simulink model "cubli_3d_model_quaternions2023"  (R2023a)
settings: Solver=ode4  StartTime=0.0  StopTime=10  FixedStep=0.01  RelTol=1e-3
InitFcn:
  | cubli_3d_model_quaternion_init
values from neighbouring files (symbols this model uses):
  b = 0    [cubli_3d_model_quaternion_init.m]
  bw = 1.06e-5    (= 1.06e-05)    [cubli_3d_model_quaternion_init.m]
  g = [0;0;9.81]    [cubli_3d_model_quaternion_init.m]
  GAMMA = [1 1 -1 0; 1 -1 0 1; -1 0 -1 1; 0 1 1 1]    [cubli_3d_model_quaternion_init.m]
  Ic_line = (Is_O + Iw1_O + Iw2_O + Iw3_O) - Iw    [cubli_3d_model_quaternion_init.m]
  invV = [0 0 0 1; 0 0 1 0; 0 -1 0 0; -1 0 0 0]    [cubli_3d_model_quaternion_init.m]
  Iw = [Iw_xx 0 0; 0 Iw_xx 0; 0 0 Iw_xx]    [cubli_3d_model_quaternion_init.m]
  l = 0.15    [cubli_3d_model_quaternion_init.m]
  mc_line = ms + 2*mw    (= 0.7)    [cubli_3d_model_quaternion_init.m]
  qs_init = [sqrt(2/3*(3-sqrt(3)))/2, -sqrt(1/3*(3+sqrt(3)))/2, sqrt(1/3*(3+sqrt(3)))/2, 0]'    [cubli_3d_model_quaternion_init.m]
  tauc = 2.46e-3    (= 0.00246)    [cubli_3d_model_quaternion_init.m]
libraries: simulink x1, matrix_library x1
settings Model: Creator=dozav  LastModifiedBy=dozav
settings RTWCC: GPUComputeCapability=5.0
settings ConfigComp: CovBoundaryAbsTol=1.0e-5

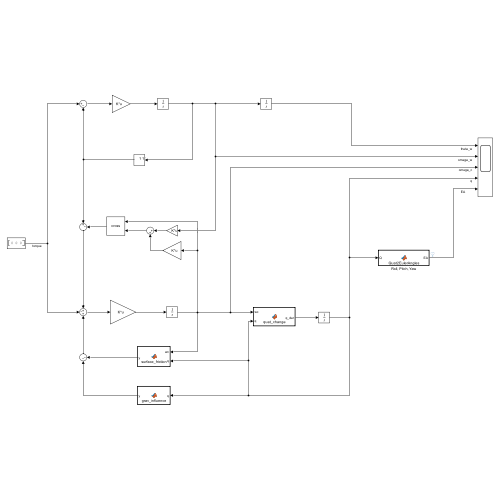
[thumbnail: Simulink's stored preview of the top-level diagram]
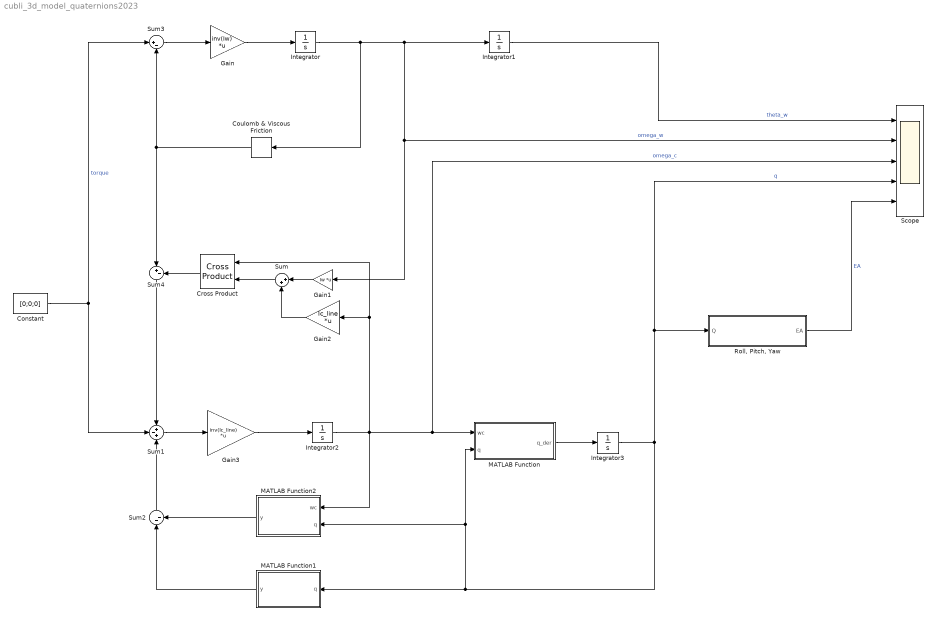
== system cubli_3d_model_quaternions2023 ==
  Constant : Constant  Value=[0;0;0]
  Coulomb & Viscous Friction : simulink/Discontinuities/Coulomb & Viscous Friction  offset=[tauc tauc tauc]  gain=[bw bw bw]
  Cross Product : matrix_library/Cross Product
  Gain : Gain  Gain=inv(Iw)  Multiplication=Matrix(K*u)
  Gain1 : Gain  Gain=Iw  Multiplication=Matrix(K*u)
  Gain2 : Gain  Gain=Ic_line  Multiplication=Matrix(K*u)
  Gain3 : Gain  Gain=inv(Ic_line)  Multiplication=Matrix(K*u)
  Integrator : Integrator  InitialCondition=[0; 0; 0]
  Integrator1 : Integrator  InitialCondition=[0; 0; 0]
  Integrator2 : Integrator  InitialCondition=[0; 0; 0]
  Integrator3 : Integrator  InitialCondition=qs_init
  MATLAB Function : MATLAB Function  TreatAsAtomicUnit=on
  MATLAB Function1 : MATLAB Function  TreatAsAtomicUnit=on
  MATLAB Function2 : MATLAB Function  TreatAsAtomicUnit=on
  "Roll, Pitch, Yaw" : MATLAB Function  TreatAsAtomicUnit=on
  Scope : Scope  NumInputPorts=5
  Sum : Sum  Inputs=|++
  Sum1 : Sum  Inputs=+-+
  Sum2 : Sum  Inputs=|--
  Sum3 : Sum  Inputs=|+-
  Sum4 : Sum  Inputs=|+-
  wires:
  Gain/1 -> Integrator/1
  Gain1/1 -> Sum/1
  Gain2/1 -> Sum/2
  Sum/1 -> Cross Product/2
  Integrator2/1 -> MATLAB Function2/1(wc), Gain2/1, Cross Product/1, Scope/3, MATLAB Function/1(wc)  "omega_c"
  Gain3/1 -> Integrator2/1
  Sum1/1 -> Gain3/1
  Constant/1 -> Sum3/1, Sum1/2  "torque"
  Sum2/1 -> Sum1/3
  Sum3/1 -> Gain/1
  Cross Product/1 -> Sum4/2
  Sum4/1 -> Sum1/1
  Integrator3/1 -> "Roll, Pitch, Yaw"/1(Q), Scope/4, MATLAB Function/2(q), MATLAB Function2/2(q), MATLAB Function1/1(q)  "q"
  MATLAB Function/1(q_der) -> Integrator3/1
  MATLAB Function1/1(y) -> Sum2/1
  Integrator/1 -> Coulomb & Viscous Friction/1, Gain1/1, Scope/2, Integrator1/1  "omega_w"
  Integrator1/1 -> Scope/1  "theta_w"
  Coulomb & Viscous Friction/1 -> Sum3/2, Sum4/1
  MATLAB Function2/1(y) -> Sum2/2
  "Roll, Pitch, Yaw"/1(EA) -> Scope/5  "EA"

== matlab function cubli_3d_model_quaternions2023/MATLAB Function1 ==
  data: q input; y output; GAMMA parameter; l parameter; g parameter; mc_line parameter
function y = grav_influence(q, GAMMA, l, g, mc_line)
%#codegen

q_skew = [0 -q(4) q(3); q(4) 0 -q(2); -q(3) q(2) 0];
G = [-q(2:4) q(1)*eye(3,3)-q_skew];

y = mc_line*9.81*l*(G*GAMMA*q);

== matlab function cubli_3d_model_quaternions2023/MATLAB Function ==
  data: wc input; q input; q_der output
function q_der = quat_change(wc, q)
%#codegen

q_skew = [0 -q(4) q(3); q(4) 0 -q(2); -q(3) q(2) 0];
G = [-q(2:4) q(1)*eye(3,3)-q_skew];

q_der = 1/2*G'*wc;

== matlab function cubli_3d_model_quaternions2023/MATLAB Function2 ==
  data: wc input; q input; y output; invV parameter; b parameter
function y = surface_friction(wc, q, invV, b)
%#codegen

q_skew = [0 -q(4) q(3); q(4) 0 -q(2); -q(3) q(2) 0];
G = [-q(2:4) q(1)*eye(3,3)-q_skew];




y = b*(G*invV*q*(G*invV*q)')*wc;

== matlab function cubli_3d_model_quaternions2023/Roll, Pitch, Yaw ==
  settings: sampleTime=0.1
  data: Q input; EA output
function EA  = Quat2EulerAngles(Q)

% Q = normr(Q);

% q0 = Q(1);
% q1 = Q(2);
% q2 = Q(3);
% q3 = Q(4);
% 
% EA = [atan2d(-2*(q2.*q3 - q1.*q0), q0.^2 - q1.^2 - q2.^2 + q3.^2), ...
%     asind(2*(q1.*q3 + q2.*q0)), ...
%     atan2d(-2*(q1.*q2 - q3.*q0), q0.^2 + q1.^2 - q2.^2 - q3.^2)];

Q = Q/norm(Q);

qw = Q(1);
qx = Q(2);
qy = Q(3);
qz = Q(4);

EA = [atan2d(2*(qw*qx+qy*qz),1-2*(qx^2+qy^2)); asind(2*(qw*qy-qx*qz)); atan2d(2*(qw*qz+qx*qy),1-2*(qy^2+qz^2))];


if ~isreal(EA)
    EA = real(EA);
end

end
